simulink model "animation"  (R2018a)
settings: Solver=VariableStepAuto  StartTime=0.0  StopTime=10.0  RelTol=1e-3
libraries: realtime_pacer_lib x1
settings Model: Creator=Sven  LastModifiedBy=Sven
settings CodeAppCC: StateflowObjectComments=on

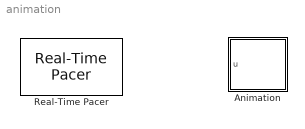
== system animation ==
  Animation : Subsystem  mask(Pendulum plot){}
      mask help: Pendulum plot
      mask Help: Pendulum animation function using Handle graphics.
      mask Display: plot([-10 10],[0 0],[-2 -2 2 2],[0 1 1 0],[0 3],[1 5])
  Real-Time Pacer : realtime_pacer_lib/Real-Time Pacer  simTimePerRealTime=1

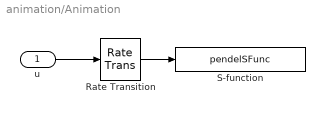
== system animation/Animation ==
  u : Inport
  Rate Transition : RateTransition
  S-function : S-Function  FunctionName=pendelSFunc  SFunctionDeploymentMode=off  EnableBusSupport=off
      settings: DeleteFcn=pendan([],[],[],'DeleteBlock');
  wires:
  u/1 -> Rate Transition/1
  Rate Transition/1 -> S-function/1
